simulink model "fxpdemo_code_only"  (Simulink 5.0)
settings: Solver=FixedStepDiscrete  SolverMode=SingleTasking  StartTime=0.0  StopTime=4-2*tsamp  FixedStep=tsamp  RelTol=1e-3  AbsTol=1e-6
PreLoadFcn:
  | preload_feedback
values from neighbouring files (symbols this model uses):
  dden = [ ... (first row only)    [preload_feedback.m]
  tsamp = 0.01    [preload_feedback.m]
libraries: fixpt_lib_4 x4
settings Model: ExecutionOrder=on  CovMetricSettings=d  Creator=andyb  LastModifiedBy=andyb  ExtModeMexFile=no_ext_comm  ExtModeTrigMode=oneshot  ExtModeArmWhenConnect=off  ExtModeAutoUpdateStatusClock=off  SaveTime=off  SaveOutput=off  LimitDataPoints=off  IntegerOverflowMsg=none  ParameterDowncastMsg=warning  ParameterOverflowMsg=warning  ParameterPrecisionLossMsg=none  RTWInlineParameters=on  RTWSystemTargetFile=ert.tlc  RTWTemplateMakefile=ert_default_tmf  RTWGenerateCodeOnly=on  RTWOptions="-aCombineOutputUpdateFcns=1 -aEnforceIntegerDowncast=1 -aExtMode=0 -aExtModeTesting=0 -aFoldNonRolledExpr=1 -aForceParamTrailComments=0 -aGenFloatMathFcnCalls=\"ANSI_C\" -aGenerateASAP2=0 -aGenerateComments=0 -aGenerateErtSFunction=0 -aGenerateReport=1 -aGenerateSampleERTMain=0 -aIgnoreCustomStorageClasses=0 -aIncDataTypeInIds=0 -aIncHierarchyInIds=0 -aIncludeMdlTerminateFcn=0 -aInitFltsAndDblsToZero=0 -aInlineInvariantSignals=1 -aInlineParameters=1 -aInlinedParameterPlacement=\"Hierarchical\" -aInlinedPrmAccess=\"Literals\" -aInsertBlockDesc=0 -aLocalBlockOutputs=1 -aMatFileLogging=0 -aMaxRTWIdLen=31 -aMultiInstanceERTCode=0 -aMultiInstanceErrorCode=\"Error\" -aPrefixModelToSubsysFcnNames=0 -aPurelyIntegerCode=1 -aRTWVerbose=1 -aRollThreshold=5 -aShowEliminatedStatements=0 -aSuppressErrorStatus=1 -aTargetOS=\"BareBoardExample\" -aZeroExternalMemoryAtStartup=0 -aZeroInternalMemoryAtStartup=0"

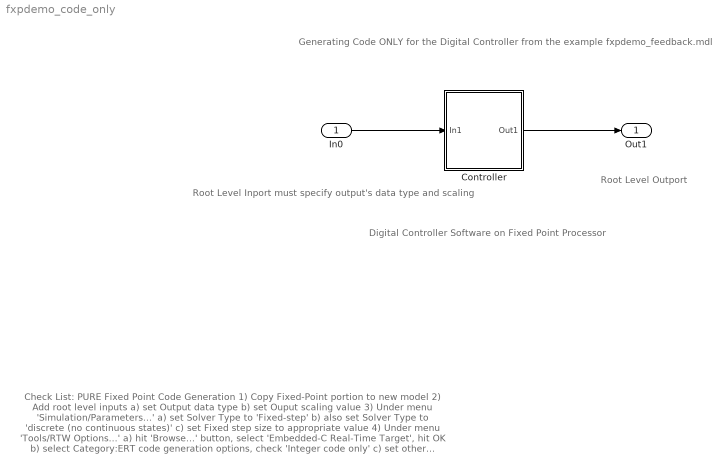
== system fxpdemo_code_only ==
  note: Root Level Inport
      | must specify output's
      | data type and scaling
  note: Generating Code ONLY for the Digital Controller
      | from the example fxpdemo_feedback.mdl
  note: Check List: PURE Fixed Point Code Generation
      |
      | 1) Copy Fixed-Point portion to new model
      |
      | 2) Add root level inputs
      |      a) set Output data type
      |      b) set Ouput scaling value
      |
      | 3) Under menu 'Simulation/Parameters...'
      |      a) set Solver Type to 'Fixed-step'
      |      b) also set Solver Type to 'discrete (no continuous states)'
      |      c) set Fixed step size to appropriate value
      |
      | 4) Under menu 'Tools/RTW Options...'
      |      a) hit 'Browse...' button, select 'Embedded-C Real-Time Target', hit OK
      |      b) select Category:ERT code generation options, check 'Integer code only'
      |      c) set other optimizations, such as inlining, as suitable...
  note: Root Level Outport
  note: Digital Controller
      | Software on
      | Fixed Point
      | Processor
  In0 : Inport  ShowAdditionalParam=on  DataType=Specify via dialog  OutDataType=sfix(8)  OutScaling=2^-4  Interpolate=off
  Controller : Subsystem
  Out1 : Outport
  wires:
  Controller/1(Out1) -> Out1/1
  In0/1 -> Controller/1(In1)

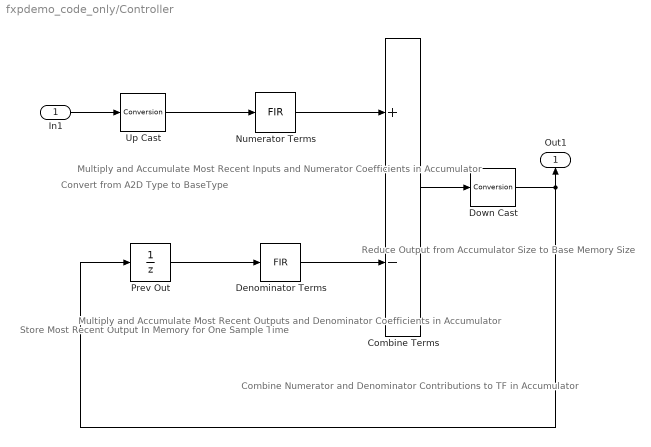
== system fxpdemo_code_only/Controller ==
  note: Reduce Output from
      | Accumulator Size to
      | Base Memory Size
  note: Combine Numerator
      | and Denominator
      | Contributions to TF
      | in Accumulator
  note: Store Most
      | Recent Output
      | In Memory for
      | One Sample Time
  note: Multiply and Accumulate
      | Most Recent Outputs and
      | Denominator Coefficients
      | in Accumulator
  note: Multiply and Accumulate
      | Most Recent Inputs and
      | Numerator Coefficients
      | in Accumulator
  note: Convert from
      | A2D Type
      | to BaseType
  In1 : Inport
  Combine Terms : Sum  Inputs=+-  ShowAdditionalParam=on  OutDataTypeMode=Specify via dialog  OutDataType=AccumType  OutScaling=2^(-28)  SaturateOnIntegerOverflow=on
  Denominator Terms : fixpt_lib_4/Filters/FIR  mgainval=dden(2:length(dden))  vinit=0.0  samptime=tsamp  GainDataTypeScalingMode=Specify via dialog  GainDataType=BaseType  GainScaling=2^-14  MatRadixGroup=Best Precision: Element-wise  OutputDataTypeScalingMode=Specify via dialog  OutDataType=AccumType  OutScaling=2^(-27)  DoSatur=on
  Down Cast : fixpt_lib_4/Data Type/Conversion  ConvertRealWorld=Real World Value  OutputDataTypeScalingMode=Specify via dialog  OutDataType=BaseType  OutScaling=2^(-12)  DoSatur=on
  Numerator Terms : fixpt_lib_4/Filters/FIR  mgainval=dnum  vinit=0.0  samptime=tsamp  GainDataTypeScalingMode=Specify via dialog  GainDataType=BaseType  GainScaling=2^-14  MatRadixGroup=Best Precision: Element-wise  OutputDataTypeScalingMode=Specify via dialog  OutDataType=AccumType  OutScaling=2^(-28)  DoSatur=on
  Prev Out : UnitDelay  X0=0.0  SampleTime=tsamp
  Up Cast : fixpt_lib_4/Data Type/Conversion  ConvertRealWorld=Real World Value  OutputDataTypeScalingMode=Specify via dialog  OutDataType=BaseType  OutScaling=2^(-12)  DoSatur=on
  Out1 : Outport  Orientation=up  InitialOutput=0
  wires:
  In1/1 -> Up Cast/1
  Up Cast/1 -> Numerator Terms/1
  Prev Out/1 -> Denominator Terms/1
  Down Cast/1 -> Out1/1, Prev Out/1
  Numerator Terms/1 -> Combine Terms/1
  Denominator Terms/1 -> Combine Terms/2
  Combine Terms/1 -> Down Cast/1
